simulink model "Integrador_RL"  (R2021a)
settings: Solver=VariableStepAuto  StartTime=0.0  StopTime=40.0  RelTol=1e-3
settings Model: Creator=Santiago  LastModifiedBy=Santiago

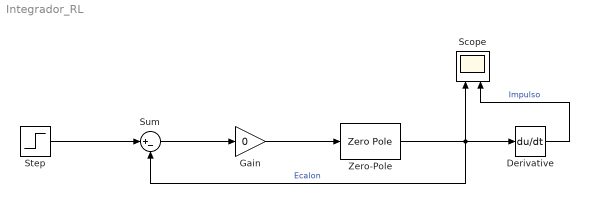
== system Integrador_RL ==
  Derivative : Derivative
  Gain : Gain  Gain=0
  Scope : Scope  NumInputPorts=2
  Step : Step  SampleTime=0
  Sum : Sum  Inputs=|+-
  Zero-Pole : ZeroPole  Zeros=[]  Poles=[0 0 0 0]
  wires:
  Step/1 -> Sum/1
  Sum/1 -> Gain/1
  Gain/1 -> Zero-Pole/1
  Zero-Pole/1 -> Sum/2, Derivative/1, Scope/1  "Ecalon"
  Derivative/1 -> Scope/2  "Impulso"
